simulink model "power_pmmotor_para_SA_Openloop"  (R2015b)
settings: Solver=ode23tb  SolverMode=SingleTasking  StartTime=0.0  StopTime=5  RelTol=1e-5
InitFcn:
  | global R;
  | R = 2.875;
  | global L;
  | L = 0.00153;
  | SampleT = 1e-4;
  | R0 = 1.5;
  | L0 = 2e-3;
  | Beta1 = 10000;
  | Beta2 = 50000;
libraries: powerlib x5, powerlib_meascontrol x1
Description:
  | Copyright 2008-2015 The MathWorks, Inc.
settings Model: ExtModeTrigMode=oneshot  ExtModeArmWhenConnect=off  ExtModeAutoUpdateStatusClock=off  Creator=MathWorks  LastModifiedBy=jxlllx
settings SolverCC: ZeroCrossAlgorithm=Adaptive
settings DataIOCC: ExternalInput=[]  LimitDataPoints=off  SaveFormat=Array  SignalLoggingSaveFormat=ModelDataLogs  SaveOutput=off  SaveTime=off  SignalLoggingName=sigsOut
settings OptimizationCC: BlockReduction=off  BooleanDataType=off  ExpressionDepthLimit=2147483647  InitFltsAndDblsToZero=on  EfficientMapNaN2IntZero=off
settings DebuggingCC: UnderspecifiedInitializationDetection=Classic  MergeDetectMultiDrivingBlocksExec=none  CheckExecutionContextPreStartOutputMsg=on  CheckExecutionContextRuntimeOutputMsg=on  SignalResolutionControl=TryResolveAllWithWarning  MultiTaskDSMMsg=warning  MultiTaskCondExecSysMsg=none  SigSpecEnsureSampleTimeMsg=none  FcnCallInpInsideContextMsg=UseLocalSettings  StateNameClashWarn=warning
settings HardwareCC: ProdBitPerPointer=32  ProdLargestAtomicFloat=None  ProdIntDivRoundTo=Undefined  ProdEndianess=Unspecified  ProdWordSize=32  ProdHWDeviceType=32-bit Generic  TargetBitPerPointer=64  TargetLongLongMode=on  TargetIntDivRoundTo=Zero  TargetEndianess=LittleEndian  TargetWordSize=64  TargetHWDeviceType=MATLAB Host  ProdEqTarget=off
settings GRTTargetCC: GeneratePreprocessorConditionals=Disable all  CombineOutputUpdateFcns=off  GRTInterface=on
settings ConfigComp: CovModelRefEnable=Off  CovSFcnEnable=off

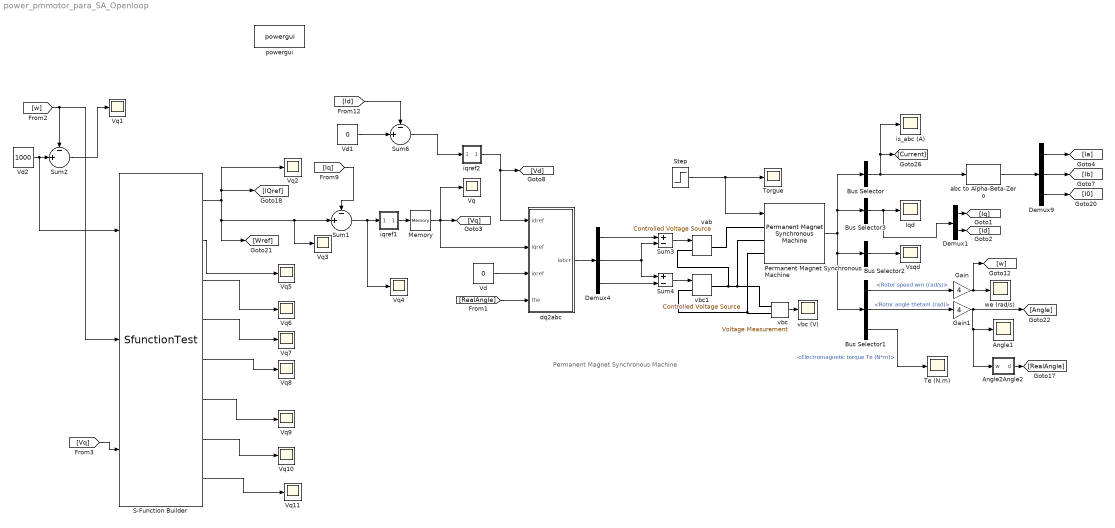
== system power_pmmotor_para_SA_Openloop ==
  note: Permanent Magnet Synchronous Machine
  Angle1 : Scope
  Angle2Angle2 : Subsystem
  Bus Selector : BusSelector  OutputSignals=Stator current is_a (A),Stator current is_b (A),Stator current is_c (A)  OutputAsBus=on
  Bus Selector1 : BusSelector  OutputSignals=Rotor speed wm (rad/s),Rotor angle thetam (rad),Electromagnetic torque Te (N*m)
  Bus Selector2 : BusSelector  OutputSignals=Stator voltage Vs_q (V),Stator voltage Vs_d (V)  OutputAsBus=on
  Bus Selector3 : BusSelector  OutputSignals=Stator current is_q (A),Stator current is_d (A)  OutputAsBus=on
  Demux1 : Demux  Outputs=2
  Demux4 : Demux  Outputs=3
  Demux9 : Demux  Outputs=3
  Gain : Gain  Gain=4  SaturateOnIntegerOverflow=on  OutDataTypeStr=Inherit: Same as input  ParamDataTypeStr=Inherit: Same as input
  Gain1 : Gain  Gain=4  SaturateOnIntegerOverflow=on  OutDataTypeStr=Inherit: Same as input  ParamDataTypeStr=Inherit: Same as input
  "Iqd " : Scope
  Memory : Memory
  Permanent Magnet Synchronous Machine : powerlib/Machines/Permanent Magnet Synchronous Machine  NbPhases=3  FluxDistribution=Sinusoidal  RotorType=Round  MechanicalLoad=Torque Tm  PresetModel=No  ShowDetailedParameters=on  MeasurementBus=off  Resistance=2.875  Inductance=8.5e-3  dqInductances=[7.2e-3,7.2e-3]  La=0.00153  MachineConstant=Flux linkage established by magnets (V.s)  Flux=0.175  VoltageCst=126.966  TorqueCst=1.05  Flat=120  Mechanical=[ 0.8,1, 4,1]  PolePairs=4  InitialConditions=[0,0, 0,0]  InitialConditions5ph=[0 0 0 0 0 0]  TsPowergui=0  TsBlock=-1  RefAngle=Aligned with phase A axis (original Park)
  S-Function Builder : S-Function  InitFcn=try, set_param(gcb,'FunctionName','SfunctionTest'), end  FunctionName=SfunctionTest  Parameters=0  SFunctionModules=SfunctionTest_wrapper SfunctionAllocateTest PID L1Adaptive  SFunctionDeploymentMode=off  EnableBusSupport=off  mask(S-Function Builder){}
      mask help: Simulink:masks:SFunctionBuilder_MD
      mask init:
      | val = [[.9  0.75 0.75 1 1 .9 .9 1]',[1 1 0.75 0.75 .9 .9 1 .9]'];try , sys = get_param(gcb,'SfunBuilderFcnName');if isempty(sys), sys = get_param(gcb,'FunctionName'); end,catch, sys = get_param(gcb,'FunctionName'); end
      settings: CopyFcn=set_param(gcbh,'LinkStatus','none')  PreSaveFcn=try, set_param(gcb,'FunctionName','SfunctionTest'), end  OpenFcn=sfunctionwizard(gcbh)
      mask Display: plot(val(:,1),val(:,2)),disp(sys), port_label('input',1,'u0'), port_label('input',2,'u1'), port_label('input',3,'u2'), port_label('output',1,'Iref'), port_label('output',2,'Xest'), port_label('output',3,'Uad'), port_label('output',4,'Um'), port_label('output',5,'RefErr'), port_label('output',6,'ThetaEst'), port_label('output',7,'StateErr'), port_label('output',8,'X')
  Step : Step  Time=0  After=0  SampleTime=0
  Sum1 : Sum  Inputs=-|+||
  Sum2 : Sum  Inputs=-|+||
  Sum3 : Sum  Inputs=+-  SaturateOnIntegerOverflow=on  InputSameDT=on  OutDataTypeStr=Inherit: Same as first input
  Sum4 : Sum  Inputs=+-  SaturateOnIntegerOverflow=on  InputSameDT=on  OutDataTypeStr=Inherit: Same as first input
  Sum6 : Sum  Inputs=-|+||
  Te (N.m) : Scope
  Torgue : Scope
  Vd : Constant  Value=0
  Vd1 : Constant  Value=0
  Vd2 : Constant  Value=1000
  Vq{,1..11} (12 alike) : Scope
  Vsqd : Scope
  abc to Alpha-Beta-Zero : powerlib_meascontrol/Transformations/abc to Alpha-Beta-Zero
  dq2abc : Subsystem
  iqref1 : Subsystem  mask(PI Controller){I=10, P=0.1, sat=[-3000, 3000]}
      mask prompts: I "Integral"; P "Proportional:"; sat "Minimum and maximum outputs:"
      mask init:
      | min=sat(1);max=sat(2);
      mask Display: disp('PI')
  iqref2 : Subsystem  mask(PI Controller){I=10, P=0.1, sat=[-3000, 3000]}
      mask prompts: I "Integral"; P "Proportional:"; sat "Minimum and maximum outputs:"
      mask init:
      | min=sat(1);max=sat(2);
      mask Display: disp('PI')
  is_abc (A) : Scope
  powergui : powerlib/powergui  SimulationMode=Continuous  SolverType=Tustin  SampleTime=0  frequency=60  SPID=on  DisableSnubberDevices=off  DisableRonSwitches=off  DisableVfSwitches=off  SwTol=0  DisplayEquations=off  Interpol=off  ExternalGateDelay=off  methode=off  Ts=0  FunctionMessages=off  echomessages=off  HookPort=off  EnableUseOfTLC=off  x0status=blocks  frequencyindice=0  Pbase=100e6  ErrMax=1e-4  Iterations=50  UnitsV=kV  UnitsW=MW  buscounter=0  RestoreLinks=warning  ResistiveCurrentMeasurement=off  Frange=[0:2:500]  Ylog=off  Xlog=on  ShowGrid=off  save=off  variable=ZData  structure=0  ZoomFFT=on  StartTime=0.0  cycles=1  DisplayStyle=1  fundamental=60  FreqAxis=off  MaxFrequency=1000  frequencyindicesteady=1  RmsSteady=1  display=off
  vab : powerlib/Electrical Sources/Controlled Voltage Source  Description=source block  Initialize=on  Source_Type=DC  Amplitude=0  Phase=0  Frequency=0  Measurements=None
      settings: AttributesFormatString=\n
  vbc : powerlib/Measurements/Voltage Measurement  Tag=PoWeRsYsTeMmEaSuReMeNt  PhasorSimulation=off  OutputType=Magnitude  PSBequivalent=0
  vbc (V) : Scope
  vbc1 : powerlib/Electrical Sources/Controlled Voltage Source  Description=source block  Initialize=on  Source_Type=DC  Amplitude=0  Phase=0  Frequency=0  Measurements=None
      settings: AttributesFormatString=\n
  we (rad/s) : Scope
  wires:
  Bus Selector1/3 -> Te (N.m)/1  "<Electromagnetic torque Te (N*m)>"
  Gain/1 -> we (rad/s)/1, [w]
  Permanent Magnet Synchronous Machine/1 -> Bus Selector1/1, Bus Selector2/1, Bus Selector3/1, Bus Selector/1
  vbc/1 -> vbc (V)/1
  Bus Selector/1 -> is_abc (A)/1, [Current], abc to Alpha-Beta-Zero/1
  Bus Selector1/1 -> Gain/1  "<Rotor speed wm (rad/s)>"
  Bus Selector1/2 -> Gain1/1  "<Rotor angle thetam (rad)>"
  Demux4/1 -> Sum3/1
  Demux4/3 -> Sum4/2
  Sum3/1 -> vab/1
  Sum4/1 -> vbc1/1
  Demux4/2 -> Sum4/1, Sum3/2
  Bus Selector2/1 -> Vsqd/1
  Bus Selector3/1 -> Demux1/1, "Iqd "/1
  Demux9/1 -> [Ia]
  Demux9/2 -> [Ib]
  Step/1 -> Permanent Magnet Synchronous Machine/1, Torgue/1
  Memory/1 -> dq2abc/2(iqref), Vq/1, [Vq]
  Gain1/1 -> Angle2Angle2/1(w), Angle1/1, [Angle]
  dq2abc/1(iabcr) -> Demux4/1
  abc to Alpha-Beta-Zero/1 -> Demux9/1
  Demux9/3 -> [I0]
  Angle2Angle2/1(d) -> [RealAngle]
  [Vq] -> S-Function Builder/3
  Sum1/1 -> iqref1/1(In_1), Vq4/1
  [Iq] -> Sum1/1
  Vd1/1 -> Sum6/2
  [Id] -> Sum6/1
  Vd/1 -> dq2abc/3(ioref)
  [RealAngle] -> dq2abc/4(the)
  S-Function Builder/1 -> Vq2/1, [IQref], [Wref], Vq3/1, Sum1/2
  Vd2/1 -> S-Function Builder/1, Sum2/2
  [w] -> S-Function Builder/2, Sum2/1
  Sum2/1 -> Vq1/1
  Demux1/1 -> [Iq]
  Demux1/2 -> [Id]
  Sum6/1 -> iqref2/1(In_1)
  iqref2/1(Out_1) -> [Vd], dq2abc/1(idref)
  S-Function Builder/2 -> Vq5/1
  S-Function Builder/4 -> Vq7/1
  S-Function Builder/3 -> Vq6/1
  S-Function Builder/5 -> Vq8/1
  iqref1/1(Out_1) -> Memory/1
  S-Function Builder/6 -> Vq9/1
  S-Function Builder/7 -> Vq10/1
  S-Function Builder/8 -> Vq11/1
  connections:
  vab/RConn1 -- Permanent Magnet Synchronous Machine/LConn1
  vbc1/RConn1 -- vbc/LConn1 -- Permanent Magnet Synchronous Machine/LConn2 -- vab/LConn1
  vbc1/LConn1 -- Permanent Magnet Synchronous Machine/LConn3 -- vbc/LConn2

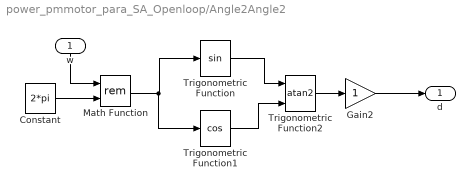
== system power_pmmotor_para_SA_Openloop/Angle2Angle2 ==
  w : Inport
  Constant : Constant  Value=2*pi
  Gain2 : Gain
  Math Function : Math  Operator=rem  SaturateOnIntegerOverflow=on
  Trigonometric Function : Trigonometry
  Trigonometric Function1 : Trigonometry  Operator=cos
  Trigonometric Function2 : Trigonometry  Operator=atan2
  d : Outport
  wires:
  Constant/1 -> Math Function/2
  w/1 -> Math Function/1
  Gain2/1 -> d/1
  Math Function/1 -> Trigonometric Function1/1, Trigonometric Function/1
  Trigonometric Function2/1 -> Gain2/1
  Trigonometric Function/1 -> Trigonometric Function2/1
  Trigonometric Function1/1 -> Trigonometric Function2/2

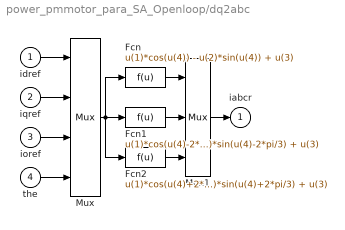
== system power_pmmotor_para_SA_Openloop/dq2abc ==
  idref : Inport
  iqref : Inport  Port=2
  ioref : Inport  Port=3
  the : Inport  Port=4
  Fcn : Fcn  Expr=u(1)*cos(u(4)) - u(2)*sin(u(4)) + u(3)
  Fcn1 : Fcn  Expr=u(1)*cos(u(4)-2*pi/3) - u(2)*sin(u(4)-2*pi/3) + u(3)
  Fcn2 : Fcn  Expr=u(1)*cos(u(4)+2*pi/3) - u(2)*sin(u(4)+2*pi/3) + u(3)
  Mux : Mux
  Mux1 : Mux  Inputs=3
  iabcr : Outport  InitialOutput=0
  wires:
  the/1 -> Mux/4
  ioref/1 -> Mux/3
  Mux/1 -> Fcn1/1, Fcn2/1, Fcn/1
  Fcn1/1 -> Mux1/2
  Fcn/1 -> Mux1/1
  Fcn2/1 -> Mux1/3
  Mux1/1 -> iabcr/1
  idref/1 -> Mux/1
  iqref/1 -> Mux/2

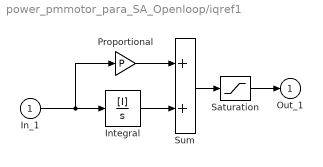
== system power_pmmotor_para_SA_Openloop/iqref1 ==
  In_1 : Inport
  Integral : TransferFcn  Numerator=[I]  Denominator=[1 0]
  Proportional : Gain  Gain=P  SaturateOnIntegerOverflow=on  OutDataTypeStr=Inherit: Same as input  ParamDataTypeStr=Inherit: Same as input
  Saturation : Saturate  UpperLimit=max  LowerLimit=min
  Sum : Sum  SaturateOnIntegerOverflow=on  InputSameDT=on  OutDataTypeStr=Inherit: Same as first input
  Out_1 : Outport  InitialOutput=0
  wires:
  Integral/1 -> Sum/2
  In_1/1 -> Integral/1, Proportional/1
  Proportional/1 -> Sum/1
  Sum/1 -> Saturation/1
  Saturation/1 -> Out_1/1

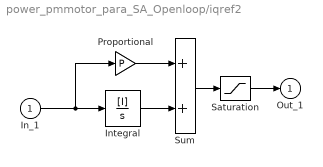
== system power_pmmotor_para_SA_Openloop/iqref2 ==
  In_1 : Inport
  Integral : TransferFcn  Numerator=[I]  Denominator=[1 0]
  Proportional : Gain  Gain=P  SaturateOnIntegerOverflow=on  OutDataTypeStr=Inherit: Same as input  ParamDataTypeStr=Inherit: Same as input
  Saturation : Saturate  UpperLimit=max  LowerLimit=min
  Sum : Sum  SaturateOnIntegerOverflow=on  InputSameDT=on  OutDataTypeStr=Inherit: Same as first input
  Out_1 : Outport  InitialOutput=0
  wires:
  Integral/1 -> Sum/2
  In_1/1 -> Integral/1, Proportional/1
  Proportional/1 -> Sum/1
  Sum/1 -> Saturation/1
  Saturation/1 -> Out_1/1
